simulink model "DualPWMRECT"  (R2021b)
settings: Solver=VariableStepAuto  StartTime=0.0  StopTime=0.5  RelTol=1e-3
libraries: spsSeriesRLCBranchLib x4, spsCurrentMeasurementLib x3, spsVoltageMeasurementLib x3, spsDiodeLib x2, spsMeanLib x2, simulink x2, spsACVoltageSourceLib x1, powerlib_extras x1, spsTHDLib x1, spsUniversalBridgeLib x1, spspowerguiLib x1, slpidlib x1
settings Model: SimulationMode=accelerator  Creator=abc6820292  LastModifiedBy=abc6820292
settings DataIOCC: ReturnWorkspaceOutputs=off

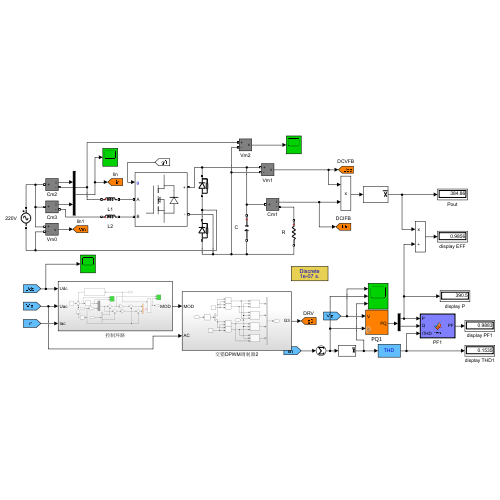
[thumbnail: Simulink's stored preview of the top-level diagram]
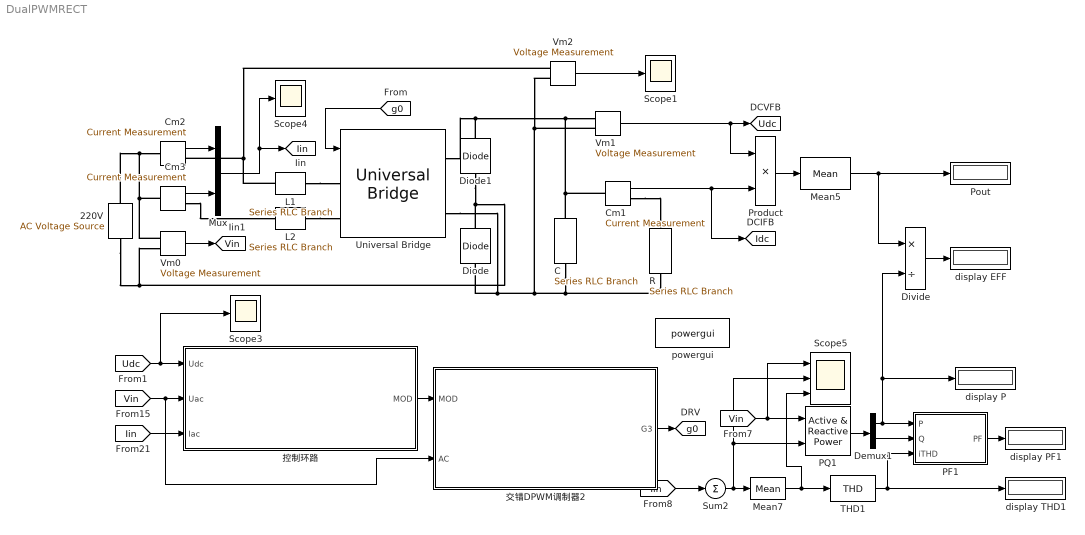
== system DualPWMRECT ==
  220V : spsACVoltageSourceLib/AC Voltage Source  Amplitude=220*1.414  Phase=0  Frequency=50  SampleTime=0  Measurements=None  BusType=swing  Pref=10e3  Qref=0  Qmin=-inf  Qmax=+inf
  C : spsSeriesRLCBranchLib/Series RLC Branch  LConnTagsString=__new0  RConnTagsString=__new0  BranchType=C  Resistance=0.01  Inductance=7e-4  SetiL0=off  InitialCurrent=0  Capacitance=1.5e-3  Setx0=on  InitialVoltage=310  Measurements=None
  Cm1 : spsCurrentMeasurementLib/Current Measurement  PhasorSimulation=off  OutputType=Complex  PSBequivalent=0
  Cm2 : spsCurrentMeasurementLib/Current Measurement  PhasorSimulation=off  OutputType=Complex  PSBequivalent=0
  Cm3 : spsCurrentMeasurementLib/Current Measurement  PhasorSimulation=off  OutputType=Complex  PSBequivalent=0
  Demux1 : Demux  Outputs=2
  Diode : spsDiodeLib/Diode  Ron=0.01  Lon=0  Vf=0.7  IC=0  UseSnubber=0  Rs=5e6  Cs=1e-8  Measurements=off
  Diode1 : spsDiodeLib/Diode  Ron=0.01  Lon=0  Vf=0.7  IC=0  UseSnubber=0  Rs=5e6  Cs=1e-8  Measurements=off
  Divide : Product  Inputs=*/
  L1 : spsSeriesRLCBranchLib/Series RLC Branch  LConnTagsString=__new0  RConnTagsString=__new0  BranchType=L  Resistance=400  Inductance=3e-4  SetiL0=off  InitialCurrent=0  Capacitance=1e-3  Setx0=off  InitialVoltage=0  Measurements=None
  L2 : spsSeriesRLCBranchLib/Series RLC Branch  LConnTagsString=__new0  RConnTagsString=__new0  BranchType=L  Resistance=400  Inductance=3e-4  SetiL0=off  InitialCurrent=0  Capacitance=1e-3  Setx0=off  InitialVoltage=0  Measurements=None
  Mean5 : spsMeanLib/Mean  Freq=50  Vinit=0  Ts=0
  Mean7 : spsMeanLib/Mean  Freq=10000  Vinit=0  Ts=0
  Mux : Mux  Inputs=2
  PF1 : MATLAB Function  TreatAsAtomicUnit=on
  PQ1 : powerlib_extras/Measurements/Active & Reactive Power  f1=50
      settings: SourceProductBaseCode=PS
  Pout : Display
      settings: Format=bank
  Product : Product
  R : spsSeriesRLCBranchLib/Series RLC Branch  LConnTagsString=__new0  RConnTagsString=__new0  BranchType=R  Resistance=200  Inductance=7e-4  SetiL0=off  InitialCurrent=0  Capacitance=1e-3  Setx0=off  InitialVoltage=0  Measurements=None
  Scope1 : Scope
  Scope3 : Scope
  Scope4 : Scope
  Scope5 : Scope  NumInputPorts=3
  Sum2 : Sum  Inputs=+
  THD1 : spsTHDLib/THD  Freq=50  Ts=0
      settings: SourceProductBaseCode=PS
  Universal Bridge : spsUniversalBridgeLib/Universal Bridge  Arms=2  SnubberResistance=1e5  SnubberCapacitance=inf  Device=MOSFET / Diodes  Ron=1e-2  Lon=0  ForwardVoltages="[  1  1  ]"  ForwardVoltage=0.7  GTOparameters=[ 10e-6 , 20e-6 ]  IGBTparameters=[ 1e-6 , 2e-6 ]  Measurements=None  Measurements_2=None  converterType=Rectifier
  Vm0 : spsVoltageMeasurementLib/Voltage Measurement  PhasorSimulation=off  OutputType=Complex  PSBequivalent=0
  Vm1 : spsVoltageMeasurementLib/Voltage Measurement  PhasorSimulation=off  OutputType=Complex  PSBequivalent=0
  Vm2 : spsVoltageMeasurementLib/Voltage Measurement  PhasorSimulation=off  OutputType=Complex  PSBequivalent=0
  display EFF : Display
  display P : Display
  display PF1 : Display
  display THD1 : Display
  powergui : spspowerguiLib/powergui  SimulationMode=Discrete  SampleTime=1e-7  frequency=60  Iterations=50  frequencyindice=0  Pbase=100e6  ErrMax=1e-4  UnitsV=kV  UnitsW=MW  buscounter=0  FunctionMessages=off  echomessages=off  EnableUseOfTLC=off  CurrentSourceSwitches=off  DisableSnubberDevices=off  DisableRonSwitches=off  DisableVfSwitches=off  DisplayEquations=off  AutomaticDiscreteSolvers=off  SolverType=Tustin/Backward Euler (TBE)  Interpol=off  ExternalGateDelay=off  methode=off  Ts=0  x0status=blocks  SPID=off  SwTol=0  HookPort=off  NonlinearTolerance=1e-4  nMaxIteration=100  ContinueOnMaxIteration=off  RestoreLinks=warning  ResistiveCurrentMeasurement=off  Frange=[0:2:500]  Ylog=off  Xlog=on  ShowGrid=off  save=off  variable=ZData  structure=QQQQQ  ZoomFFT=off  StartTime=0.5  cycles=15  DisplayStyle=1  fundamental=50  FreqAxis=off  MaxFrequency=1000  frequencyindicesteady=1  RmsSteady=1  display=off
  交错DPWM调制器2 : Subsystem
  控制环路 : Subsystem
  tag scope: Idc=global, Iin=global, Udc=global, Vin=global, g0=global
  wires:
  [Udc] -> 控制环路/1(Udc), Scope3/1
  [Iin] -> 控制环路/3(Iac)
  Vm0/1 -> [Vin]
  [Vin] -> 交错DPWM调制器2/2(AC), 控制环路/2(Uac)
  [g0] -> Universal Bridge/1
  PF1/1(PF) -> display PF1/1
  THD1/1 -> display THD1/1, PF1/3(iTHD)
  [Vin] -> Scope5/1, PQ1/1
  Demux1/1 -> Divide/2, display P/1, PF1/1(P)
  PQ1/1 -> Demux1/1
  Mean7/1 -> Scope5/3, THD1/1
  Demux1/2 -> PF1/2(Q)
  Vm2/1 -> Scope1/1
  Divide/1 -> display EFF/1
  Vm1/1 -> [Udc], Product/1
  Cm1/1 -> [Idc], Product/2
  Cm2/1 -> Mux/1
  Cm3/1 -> Mux/2
  Mux/1 -> Scope4/1, [Iin]
  控制环路/1(MOD) -> 交错DPWM调制器2/1(MOD)
  交错DPWM调制器2/1(G3) -> [g0]
  Sum2/1 -> PQ1/2, Scope5/2, Mean7/1
  [Iin] -> Sum2/1
  Product/1 -> Mean5/1
  Mean5/1 -> Pout/1, Divide/1
  connections:
  Cm1/RConn1 -- R/LConn1
  R/RConn1 -- C/RConn1 -- Diode/LConn1 -- Universal Bridge/RConn2 -- Vm2/LConn2 -- Vm1/LConn2
  220V/LConn1 -- Diode/RConn1 -- Diode1/LConn1 -- Vm0/LConn2
  Vm2/LConn1 -- L1/LConn1 -- Cm2/RConn1
  C/LConn1 -- Cm1/LConn1 -- Diode1/RConn1 -- Universal Bridge/RConn1 -- Vm1/LConn1
  220V/RConn1 -- Cm3/LConn1 -- Vm0/LConn1 -- Cm2/LConn1
  L1/RConn1 -- Universal Bridge/LConn1
  Cm3/RConn1 -- L2/LConn1
  L2/RConn1 -- Universal Bridge/LConn2

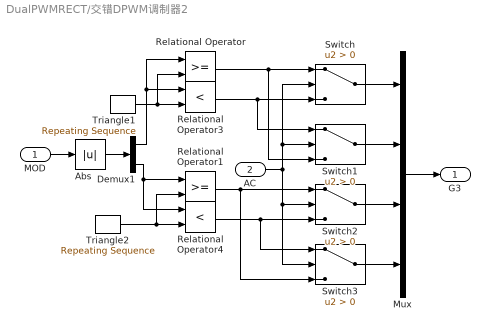
== system DualPWMRECT/交错DPWM调制器2 ==
  MOD : Inport
  AC : Inport  Port=2
  Abs : Abs
  Demux1 : Demux  Outputs=2
  Mux : Mux
  Relational Operator : RelationalOperator  OutDataTypeStr=boolean  RndMeth=Nearest
  Relational Operator1 : RelationalOperator  OutDataTypeStr=boolean  RndMeth=Nearest
  Relational Operator3 : RelationalOperator  Operator=<  OutDataTypeStr=boolean  RndMeth=Nearest
  Relational Operator4 : RelationalOperator  Operator=<  OutDataTypeStr=boolean  RndMeth=Nearest
  Switch{,1..3} (4 alike) : Switch  Criteria=u2 > Threshold
  Triangle1 : simulink/Sources/Repeating Sequence  rep_seq_t=[0 1/60000/2 1/60000]  rep_seq_y=[0 1 0]
  Triangle2 : simulink/Sources/Repeating Sequence  rep_seq_t=[0 1/60000/2 1/60000]  rep_seq_y=[1 0 1]
  G3 : Outport
  wires:
  Relational Operator1/1 -> Switch3/3, Switch2/1
  Relational Operator4/1 -> Switch3/1, Switch2/3
  Switch3/1 -> Mux/4
  Switch2/1 -> Mux/3
  Relational Operator3/1 -> Switch1/1, Switch/3
  Switch1/1 -> Mux/2
  Switch/1 -> Mux/1
  Relational Operator/1 -> Switch/1, Switch1/3
  Triangle1/1 -> Relational Operator/2, Relational Operator3/2
  Triangle2/1 -> Relational Operator1/2, Relational Operator4/2
  Mux/1 -> G3/1
  AC/1 -> Switch2/2, Switch3/2, Switch1/2, Switch/2
  Demux1/2 -> Relational Operator1/1, Relational Operator4/1
  Demux1/1 -> Relational Operator3/1, Relational Operator/1
  Abs/1 -> Demux1/1
  MOD/1 -> Abs/1

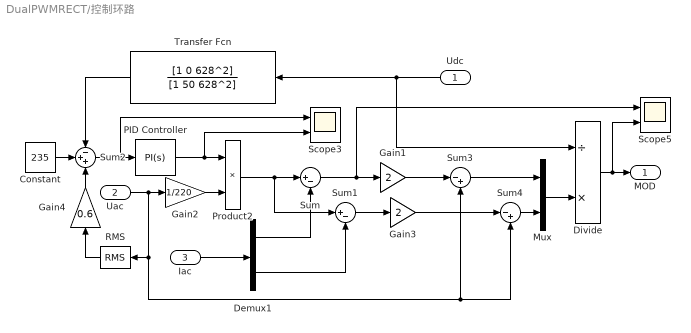
== system DualPWMRECT/控制环路 ==
  Udc : Inport
  Uac : Inport  Port=2
  Iac : Inport  Port=3
  Constant : Constant  Value=235
  Demux1 : Demux  Outputs=2
  Divide : Product  Inputs=/*
  Gain1 : Gain  Gain=2
  Gain2 : Gain  Gain=1/220
  Gain3 : Gain  Gain=2
  Gain4 : Gain  Gain=0.6
  Mux : Mux  Inputs=2
  PID Controller : slpidlib/PID Controller  Controller=PI  Form=Parallel  TimeDomain=Continuous-time  UseExternalTs=off  SampleTime=-1  IntegratorMethod=Forward Euler  FilterMethod=Forward Euler  ControllerParametersSource=internal  P=0.1  I=6  D=0.005  UseFilter=on  N=100  TunerSelectOption=Transfer Function Based (PID Tuner App)  InitialConditionSource=internal  InitialConditionForIntegrator=0  InitialConditionForFilter=0  DifferentiatorICPrevScaledInput=0  ExternalReset=none  TrackingMode=off  Kt=1  LimitOutput=on  SatLimitsSource=internal  UpperSaturationLimit=100  LowerSaturationLimit=0  LinearizeAsGain=on  AntiWindupMode=clamping  Kb=1  POutMin=[]  POutMax=[]  IOutMin=[]  IOutMax=[]  DOutMin=[]  DOutMax=[]  NOutMin=[]  NOutMax=[]  SumOutMin=[]  SumOutMax=[]  SaturationOutMin=[]  SaturationOutMax=[]  PParamMin=[]  PParamMax=[]  IParamMin=[]  IParamMax=[]  DParamMin=[]  DParamMax=[]  NParamMin=[]  NParamMax=[]  KbParamMin=[]  KbParamMax=[]  KtParamMin=[]  KtParamMax=[]  KbOutMin=[]  KbOutMax=[]  KtOutMin=[]  KtOutMax=[]  IntegratorOutMin=[]  IntegratorOutMax=[]  FilterOutMin=[]  FilterOutMax=[]  SumI1OutMin=[]  SumI1OutMax=[]  SumI2OutMin=[]  SumI2OutMax=[]  SumI3OutMin=[]  SumI3OutMax=[]  SumI4OutMin=[]  SumI4OutMax=[]  SumDOutMin=[]  SumDOutMax=[]  DifferentiatorOutMin=[]  DifferentiatorOutMax=[]  FilterDiffOutCoefMin=[]  FilterDiffOutCoefMax=[]  ReciprocalOutMin=[]  ReciprocalOutMax=[]  SumDenOutMin=[]  SumDenOutMax=[]  SumNumOutMin=[]  SumNumOutMax=[]  DivideOutMin=[]  DivideOutMax=[]  UdiffTsProdOutMin=[]  UdiffTsProdOutMax=[]  NTsProdOutMin=[]  NTsProdOutMax=[]  UintegralTsProdOutMin=[]  UintegralTsProdOutMax=[]  UngainTsProdOutMin=[]  UngainTsProdOutMax=[]  FilterDenConstantOutDataTypeStr=Inherit: Inherit via back propagation  FilterDenConstantOutMin=[]  FilterDenConstantOutMax=[]  PCopyOutDataTypeStr=Inherit: Inherit via back propagation  PCopyOutMin=[]  PCopyOutMax=[]  NCopyOutDataTypeStr=Inherit: Inherit via back propagation  NCopyOutMin=[]  NCopyOutMax=[]  IntegratorContinuousStateAttributes=''  IntegratorStateMustResolveToSignalObject=off  IntegratorRTWStateStorageClass=Auto  FilterContinuousStateAttributes=''  FilterStateMustResolveToSignalObject=off  FilterRTWStateStorageClass=Auto  ParallelPVariant=InternalParameters  IdealPVariant=Disabled  IVariant=InternalParameters  DVariant=Disabled  IntegratorVariant=Continuous  SatVariant=Enabled  AWVariant=ContClampingParallel  PCopyVariant=Disabled  TRVariant=Disabled  FdbkBlocksVariant=Forward  IdealPFdbkVariant=Disabled  SatFdbkVariant=Disabled  DerivativeFilterVariant=Disabled  NVariant=Disabled  NCopyVariant=Disabled_SignalSpec  FilterICVariant=Disabled  IntegratorICVariant=InternalICs  ExternalResetVariant=Disabled  TRSumVariant=Passthrough  SumFdbkVariant=Disabled  SumVariant=Sum_PI  TsampFilterVariant=InternalTs  TsampNgainVariant=Passthrough  TsampIntegralVariant=Passthrough  ExternalSaturationOutDataTypeStr=Inherit: Same as second input
  Product2 : Product  RndMeth=Zero
  RMS : spsRMSLib/RMS  TrueRMS=off  Freq=50  RMSInit=220  Ts=0
  Scope3 : Scope  NumInputPorts=2
  Scope5 : Scope  NumInputPorts=2
  Sum : Sum  Inputs=|+-
  Sum1 : Sum  Inputs=|+-
  Sum2 : Sum  Inputs=-++
  Sum3 : Sum  Inputs=|-+
  Sum4 : Sum  Inputs=|-+
  Transfer Fcn : TransferFcn  Numerator=[1 0 628^2]  Denominator=[1 50 628^2]
  MOD : Outport
  wires:
  Gain2/1 -> Product2/2
  PID Controller/1 -> Product2/1, Scope3/2
  Sum2/1 -> Scope3/1, PID Controller/1
  Udc/1 -> Divide/1, Transfer Fcn/1
  Sum/1 -> Gain1/1, Scope5/1
  Gain3/1 -> Sum4/1
  Gain1/1 -> Sum3/1
  Iac/1 -> Demux1/1
  Demux1/1 -> Sum/2
  Product2/1 -> Sum1/1, Sum/1
  Demux1/2 -> Sum1/2
  Sum1/1 -> Gain3/1
  Sum4/1 -> Mux/2
  Sum3/1 -> Mux/1
  Mux/1 -> Divide/2
  Constant/1 -> Sum2/2
  Transfer Fcn/1 -> Sum2/1
  Divide/1 -> Scope5/2, MOD/1
  Uac/1 -> Sum4/2, Sum3/2, RMS/1, Gain2/1
  Gain4/1 -> Sum2/3
  RMS/1 -> Gain4/1

== matlab function DualPWMRECT/PF1 ==
  data: P input; PF output; Q input; iTHD input
function PF = fcn(P,Q,iTHD)
% This block supports an embeddable subset of the MATLAB language.
% See the help menu for details. 
PF=(P/sqrt(P*P+Q*Q))/(sqrt(1+iTHD*iTHD));
